simulink model "Copy_of_Controller"  (R2023a)
settings: Solver=FixedStepDiscrete  StartTime=0.0  StopTime=inf  FixedStep=0.001  RelTol=1e-3  EnableMultiTasking=on
undefined symbols (not defined in the file or in its folder): C, den_d, Discrete, K, K_down, num_d, sys_d, sys_d_down, Time
libraries: simulink x12, quarc_library x4, eeGeneralControl x4, ctrlSharedLib x2, simulink_extras x1
settings Model: SimulationMode=external  ExtModeTrigType=signal  ExtModeTrigDuration=60000  ExtModeTrigDirection=either  ExtModeTrigLevel=0.500000  Creator=colegiusto  LastModifiedBy=colegiusto
settings SolverCC: PositivePriorityOrder=on
settings RTWCC: Description=QUARC Win64 Target Using Toolchain  SystemTargetFile=quarc_win64.tlc  Toolchain=QUARC win64 | nmake (64-bit Windows)  BuildConfiguration=Faster Runs
settings STFCustomTargetCC: TargetLangStandard=C89/C90 (ANSI)  SystemTargetFile=quarc_win64.tlc
settings GRTTargetCC: TargetLangStandard=C89/C90 (ANSI)  ParMdlRefBuildCompliant=off  CompOptLevelCompliant=off  CombineOutputUpdateFcns=off  MatFileLogging=off  CPPClassGenCompliant=off  GRTInterface=on  ExtMode=on  ExtModeMexFile=quarc_comm

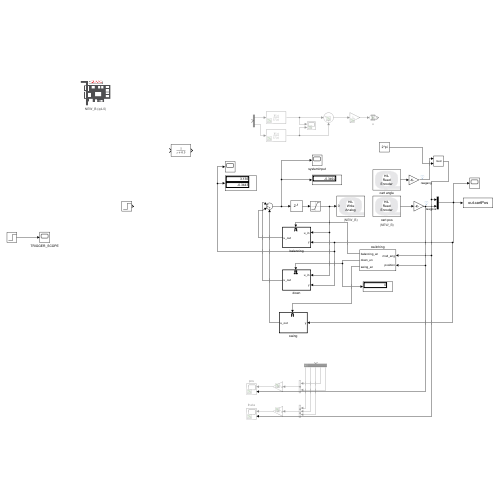
[thumbnail: Simulink's stored preview of the top-level diagram]
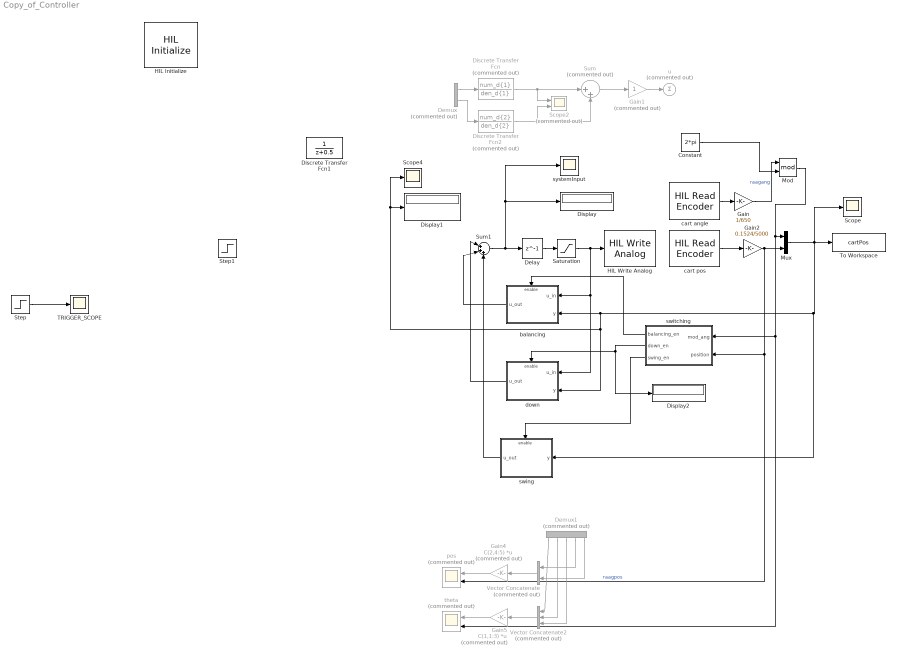
== system Copy_of_Controller ==
  Constant : Constant  Value=2*pi
  Delay : Delay  DelayLength=1
  Demux : Demux  Commented=on  Outputs=2
  Demux1 : Demux  Commented=on  Outputs=5
  Discrete Transfer Fcn : DiscreteTransferFcn  Commented=on  Numerator=num_d{1}  Denominator=den_d{1}  SampleTime=0.001
  Discrete Transfer Fcn1 : DiscreteTransferFcn
  Discrete Transfer Fcn2 : DiscreteTransferFcn  Commented=on  Numerator=num_d{2}  Denominator=den_d{2}  SampleTime=0.001
  Display : Display
  Display1 : Display
  Display2 : Display
  Gain : Gain  Gain=1/650
  Gain1 : Gain  Commented=on
  Gain2 : Gain  Gain=0.1524/5000
  Gain4 : Gain  Commented=on  Gain=C(2,4:5)  Multiplication=Matrix(K*u)
  Gain5 : Gain  Commented=on  Gain=C(1,1:3)  Multiplication=Matrix(K*u)
  HIL Initialize : quarc_library/Data Acquisition/Generic/Configuration/HIL Initialize  object_name=NEW_B  board_type=q4  board_number=0  board_options=""  exclusive=off  active=on  hardware_clocks=[0:1]  clock_modes=[0 0]  initial_clock_frequencies=[]  set_clock_params_at_start=on  set_clock_params_at_switch_in=off  set_clock_frequencies_at_start=off  set_clock_frequencies_at_switch_in=off  analog_input_channels=[0:3]  analog_input_configurations=[]  analog_input_maximums=10  analog_input_minimums=-10  set_analog_input_params_at_start=off  set_analog_input_params_at_switch_in=off  analog_output_channels=[0:3]  analog_output_maximums=[10]  analog_output_minimums=[-10]  initial_analog_outputs=[0]  final_analog_outputs=[0]  watchdog_analog_outputs=0  set_analog_output_params_at_start=on  set_analog_output_params_at_switch_in=off  set_analog_outputs_at_start=on  set_analog_outputs_at_switch_in=off  set_analog_outputs_at_terminate=on  set_analog_outputs_at_switch_out=off  set_analog_outputs_on_watchdog=off  digital_input_channels=[]  digital_output_channels=[]  digital_output_configuration=[]  initial_digital_outputs=[1]  final_digital_outputs=[1]  watchdog_digital_outputs=[2]  set_digital_output_params_at_start=off  set_digital_output_params_at_switch_in=off  set_digital_outputs_at_start=on  set_digital_outputs_at_switch_in=off  set_digital_outputs_at_terminate=on  set_digital_outputs_at_switch_out=off  set_digital_outputs_on_watchdog=off  encoder_channels=[0:3]  quadrature=[4]  encoder_filter_frequency=(1/60e-9)/1  initial_encoder_counts=[0]  set_encoder_params_at_start=on  set_encoder_params_at_switch_in=off  set_encoder_counts_at_start=on  set_encoder_counts_at_switch_in=off  pwm_channels=[]  pwm_modes=[0]  pwm_frequency=(1/60e-9)/1024  pwm_configuration=[]  pwm_alignment=[]  pwm_polarity=[]  pwm_leading_deadband=[]  pwm_trailing_deadband=[]  initial_pwm_outputs=[0]  final_pwm_outputs=[0]  watchdog_pwm_outputs=[]  set_pwm_params_at_start=on  set_pwm_params_at_switch_in=off  set_pwm_outputs_at_start=on  set_pwm_outputs_at_switch_in=off  set_pwm_outputs_at_terminate=on  set_pwm_outputs_at_switch_out=off  set_pwm_outputs_on_watchdog=off  other_output_channels=[]  initial_other_outputs=[]  final_other_outputs=[]  watchdog_other_outputs=[]  set_other_outputs_at_start=off  set_other_outputs_at_switch_in=off  set_other_outputs_at_terminate=off  set_other_outputs_at_switch_out=off  set_other_outputs_on_watchdog=off
  HIL Write Analog : quarc_library/Data Acquisition/Generic/Immediate I//O/HIL Write Analog  object_name=NEW_B  channels=0  sample_time=0.001  active=off  vector_input=off
  Mod : Math  Operator=mod
  Mux : Mux  Inputs=2
  Saturation : Saturate  UpperLimit=5  LowerLimit=-5
  Scope : Scope
  Scope2 : Scope  Commented=on  NumInputPorts=2
  Scope4 : Scope
  Step : Step  Time=0.001  SampleTime=0
  Step1 : Step  After=0.3  SampleTime=0
  Sum : Sum  Commented=on  Inputs=|++
  Sum1 : Sum  Inputs=|+++
  TRIGGER_SCOPE : Scope
  To Workspace : ToWorkspace  VariableName=cartPos  SaveFormat=Structure With Time  SampleTime=-1
  Vector Concatenate : Concatenate  Commented=on
  Vector Concatenate2 : Concatenate  Commented=on  NumInputs=3
  balancing : Subsystem
  cart angle : quarc_library/Data Acquisition/Generic/Immediate I//O/HIL Read Encoder  object_name=NEW_B  channels=3  sample_time=0.001  active=on  vector_output=on  data_type_mode=Inherit via back propagation  data_type=double
  cart pos : quarc_library/Data Acquisition/Generic/Immediate I//O/HIL Read Encoder  object_name=NEW_B  channels=2  sample_time=0.001  active=on  vector_output=on  data_type_mode=Inherit via back propagation  data_type=double
  down : Subsystem
  pos : Scope  Commented=on  NumInputPorts=2
  swing : Subsystem
  switching : Subsystem
  systemInput : Scope
  theta : Scope  Commented=on  NumInputPorts=2
  u : Sum  Commented=on  Inputs=+
  wires:
  cart angle/1 -> Gain/1
  Step/1 -> TRIGGER_SCOPE/1
  Gain/1 -> Mod/1  "raagang"
  Mux/1 -> swing/1(y), balancing/2(y), down/2(y), Scope4/1, Display1/1, To Workspace/1, Scope/1
  Saturation/1 -> balancing/1(u_in), down/1(u_in), HIL Write Analog/1
  cart pos/1 -> Gain2/1
  Gain2/1 -> Mux/2, switching/2(position), pos/2  "raagpos"
  Demux/1 -> Discrete Transfer Fcn/1
  Demux/2 -> Discrete Transfer Fcn2/1
  Sum/1 -> Gain1/1
  Discrete Transfer Fcn2/1 -> Sum/2, Scope2/2
  Discrete Transfer Fcn/1 -> Sum/1, Scope2/1
  Gain1/1 -> u/1
  Demux1/4 -> Vector Concatenate/1
  Demux1/5 -> Vector Concatenate/2
  Vector Concatenate/1 -> Gain4/1
  Demux1/1 -> Vector Concatenate2/1
  Demux1/2 -> Vector Concatenate2/2
  Demux1/3 -> Vector Concatenate2/3
  Vector Concatenate2/1 -> Gain5/1
  Gain4/1 -> pos/1
  Gain5/1 -> theta/1
  Constant/1 -> Mod/2
  Mod/1 -> theta/2, switching/1(mod_ang), Mux/1
  Delay/1 -> Saturation/1
  switching/1(balancing_en) -> balancing/Enable
  switching/2(down_en) -> Display2/1, down/Enable
  balancing/1(u_out) -> Sum1/2
  Sum1/1 -> systemInput/1, Display/1, Delay/1
  switching/3(swing_en) -> swing/Enable
  swing/1(u_out) -> Sum1/3
  down/1(u_out) -> Sum1/1

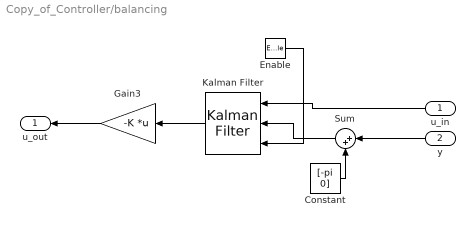
== system Copy_of_Controller/balancing ==
  u_in : Inport
  y : Inport  Port=2
  Enable : EnablePort  StatesWhenEnabling=reset  ShowOutputPort=on
  Constant : Constant  Value=[-pi 0]
  Gain3 : Gain  Gain=-K  Multiplication=Matrix(K*u)
  Kalman Filter : ctrlSharedLib/Kalman Filter  TimeDomain=Discrete-Time  UseCurrentEstimator=on  ModelSource=Individual A, B, C, D matrices  ModelSourceVariable=ss(0.95,1,1,0,1)  A=sys_d.A  B=sys_d.B  C=sys_d.C  D=sys_d.D  NumberOfStates=1  NumberOfInputs=1  NumberOfOutputs=1  InitialEstimateSource=Dialog  X0=0  P0=10  UseK=off  UseGH=off  NumberOfProcessNoiseInputs=1  G=1  TimeInvariantG=on  H=0  TimeInvariantH=on  Q=1  TimeInvariantQ=on  R=10  TimeInvariantR=on  N=0  TimeInvariantN=on  AddInputPort=on  AddEnablePort=off  ExternalReset=Rising  OutputEstimatedY=off  OutputP=off  Ts=0.001
  Sum : Sum  Inputs=|++
  u_out : Outport  OutputWhenDisabled=reset  InitialOutput=[0]
  wires:
  Kalman Filter/1 -> Gain3/1
  u_in/1 -> Kalman Filter/1
  Gain3/1 -> u_out/1
  y/1 -> Sum/1
  Constant/1 -> Sum/2
  Sum/1 -> Kalman Filter/2
  Enable/1 -> Kalman Filter/3

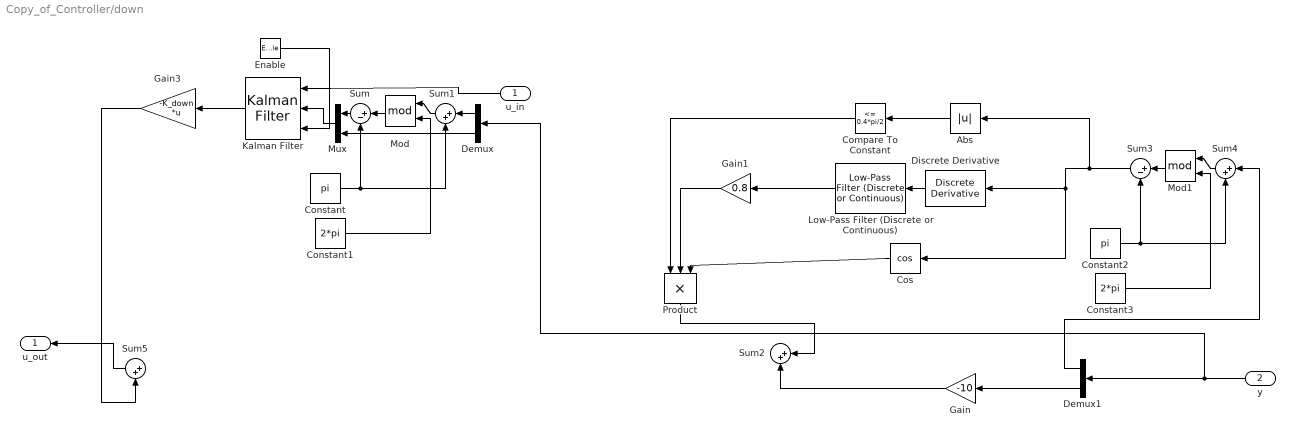
== system Copy_of_Controller/down ==
  u_in : Inport
  y : Inport  Port=2
  Enable : EnablePort  StatesWhenEnabling=reset  ShowOutputPort=on
  Abs : Abs  SaturateOnIntegerOverflow=off
  Compare To Constant : simulink/Logic and Bit Operations/Compare To Constant  relop=<=  const=0.4*pi/2  OutDataTypeStr=boolean
  Constant : Constant  Value=pi
  Constant1 : Constant  Value=2*pi
  Constant2 : Constant  Value=pi
  Constant3 : Constant  Value=2*pi
  Cos : Trigonometry  Operator=cos
  Demux : Demux  Outputs=2
  Demux1 : Demux  Outputs=2
  Discrete Derivative : simulink/Discrete/Discrete Derivative  gainval=1.0  ICPrevScaledInput=0.0  OutMin=[]  OutMax=[]  OutDataType=fixdt(1, 16)  OutScaling=2^-10  DoSatur=off
  Gain : Gain  Gain=-10
  Gain1 : Gain  Gain=0.8
  Gain3 : Gain  Gain=-K_down  Multiplication=Matrix(K*u)
  Kalman Filter : ctrlSharedLib/Kalman Filter  TimeDomain=Discrete-Time  UseCurrentEstimator=on  ModelSource=Individual A, B, C, D matrices  ModelSourceVariable=ss(0.95,1,1,0,1)  A=sys_d_down.A  B=sys_d_down.B  C=sys_d_down.C  D=sys_d_down.D  NumberOfStates=1  NumberOfInputs=1  NumberOfOutputs=1  InitialEstimateSource=Dialog  X0=0  P0=10  UseK=off  UseGH=off  NumberOfProcessNoiseInputs=1  G=1  TimeInvariantG=on  H=0  TimeInvariantH=on  Q=1  TimeInvariantQ=on  R=10  TimeInvariantR=on  N=0  TimeInvariantN=on  AddInputPort=on  AddEnablePort=off  ExternalReset=Rising  OutputEstimatedY=off  OutputP=off  Ts=0.001
  Low-Pass Filter (Discrete or Continuous) : eeGeneralControl/Low-Pass Filter (Discrete or Continuous)  K=1  T=0.01  B=inf  A=-inf  init_option=Inherited from block input  x0=0  Ts=-1
  Mod : Math  Operator=mod
  Mod1 : Math  Operator=mod
  Mux : Mux  Inputs=2
  Product : Product  Inputs=3
  Sum : Sum  Inputs=|+-
  Sum{1..2,4..5} (4 alike) : Sum  Inputs=|++
  Sum3 : Sum  Inputs=|+-
  u_out : Outport  OutputWhenDisabled=reset  InitialOutput=[0]
  wires:
  Kalman Filter/1 -> Gain3/1
  u_in/1 -> Kalman Filter/1
  Demux/2 -> Mux/2
  Mux/1 -> Kalman Filter/2
  Demux/1 -> Sum1/1
  Mod/1 -> Sum/1
  Sum1/1 -> Mod/1
  Constant/1 -> Sum1/2, Sum/2
  Constant1/1 -> Mod/2
  Sum/1 -> Mux/1
  Constant3/1 -> Mod1/2
  Product/1 -> Sum2/1
  Gain1/1 -> Product/2
  Cos/1 -> Product/3
  Sum3/1 -> Abs/1, Cos/1, Discrete Derivative/1
  Abs/1 -> Compare To Constant/1
  Demux1/2 -> Gain/1
  Gain/1 -> Sum2/2
  Constant2/1 -> Sum4/2, Sum3/2
  Demux1/1 -> Sum4/1
  Sum4/1 -> Mod1/1
  Compare To Constant/1 -> Product/1
  Discrete Derivative/1 -> Low-Pass Filter (Discrete or Continuous)/1
  Mod1/1 -> Sum3/1
  y/1 -> Demux/1, Demux1/1
  Low-Pass Filter (Discrete or Continuous)/1 -> Gain1/1
  Gain3/1 -> Sum5/2
  Sum5/1 -> u_out/1
  Enable/1 -> Kalman Filter/3

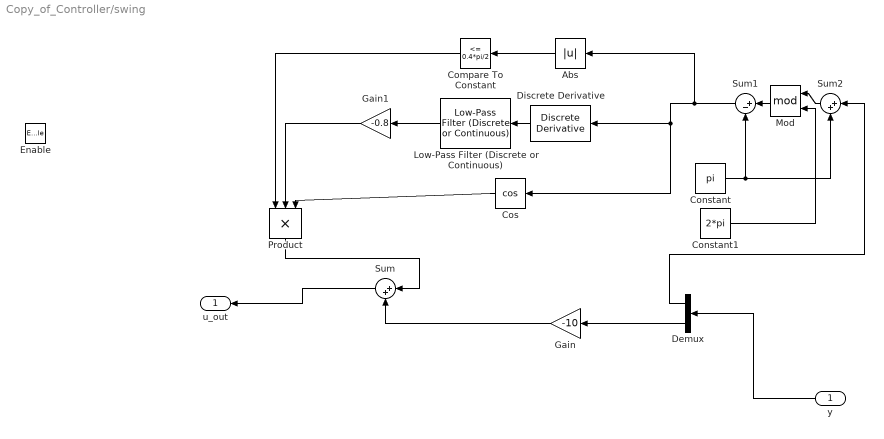
== system Copy_of_Controller/swing ==
  y : Inport
  Enable : EnablePort  StatesWhenEnabling=reset
  Abs : Abs  SaturateOnIntegerOverflow=off
  Compare To Constant : simulink/Logic and Bit Operations/Compare To Constant  relop=<=  const=0.4*pi/2  OutDataTypeStr=boolean
  Constant : Constant  Value=pi
  Constant1 : Constant  Value=2*pi
  Cos : Trigonometry  Operator=cos
  Demux : Demux  Outputs=2
  Discrete Derivative : simulink/Discrete/Discrete Derivative  gainval=1.0  ICPrevScaledInput=0.0  OutMin=[]  OutMax=[]  OutDataType=fixdt(1, 16)  OutScaling=2^-10  DoSatur=off
  Gain : Gain  Gain=-10
  Gain1 : Gain  Gain=-0.8
  Low-Pass Filter (Discrete or Continuous) : eeGeneralControl/Low-Pass Filter (Discrete or Continuous)  K=1  T=0.01  B=inf  A=-inf  init_option=Inherited from block input  x0=0  Ts=-1
  Mod : Math  Operator=mod
  Product : Product  Inputs=3
  Sum : Sum  Inputs=|++
  Sum1 : Sum  Inputs=|+-
  Sum2 : Sum  Inputs=|++
  u_out : Outport  OutputWhenDisabled=reset  InitialOutput=[0]
  wires:
  y/1 -> Demux/1
  Sum/1 -> u_out/1
  Demux/2 -> Gain/1
  Gain/1 -> Sum/2
  Demux/1 -> Sum2/1
  Discrete Derivative/1 -> Low-Pass Filter (Discrete or Continuous)/1
  Low-Pass Filter (Discrete or Continuous)/1 -> Gain1/1
  Constant/1 -> Sum2/2, Sum1/2
  Constant1/1 -> Mod/2
  Mod/1 -> Sum1/1
  Sum2/1 -> Mod/1
  Sum1/1 -> Abs/1, Cos/1, Discrete Derivative/1
  Gain1/1 -> Product/2
  Product/1 -> Sum/1
  Abs/1 -> Compare To Constant/1
  Compare To Constant/1 -> Product/1
  Cos/1 -> Product/3

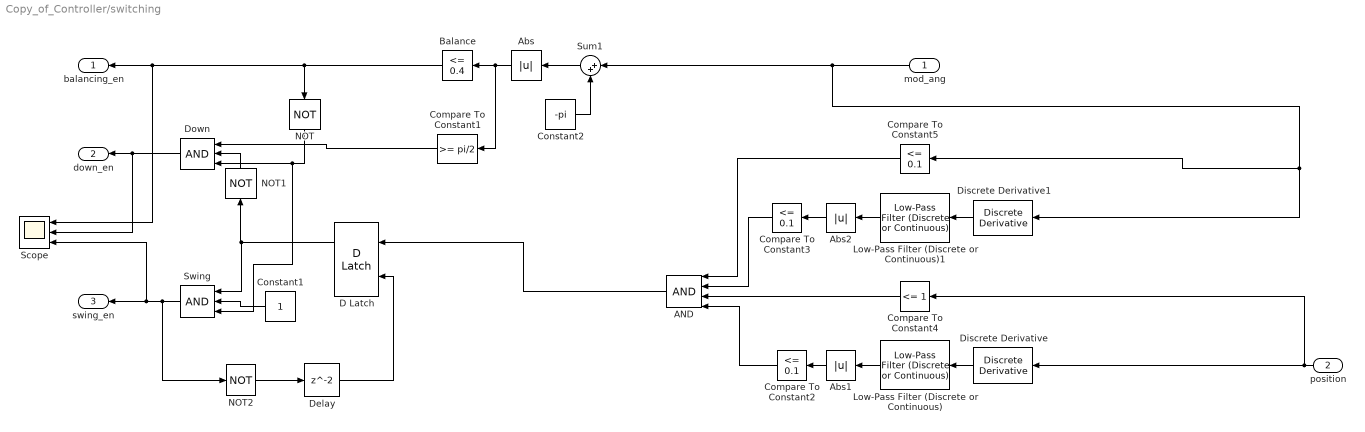
== system Copy_of_Controller/switching ==
  mod_ang : Inport
  position : Inport  Port=2
  AND : Logic  Inputs=4  IconShape=distinctive  AllPortsSameDT=off  OutDataTypeStr=boolean
  Abs : Abs  SaturateOnIntegerOverflow=off
  Abs1 : Abs  SaturateOnIntegerOverflow=off
  Abs2 : Abs  SaturateOnIntegerOverflow=off
  Balance : simulink/Logic and Bit Operations/Compare To Constant  relop=<=  const=0.4  OutDataTypeStr=boolean
  Compare To Constant1 : simulink/Logic and Bit Operations/Compare To Constant  relop=>=  const=pi/2  OutDataTypeStr=boolean
  Compare To Constant2 : simulink/Logic and Bit Operations/Compare To Constant  relop=<=  const=0.1  OutDataTypeStr=boolean
  Compare To Constant3 : simulink/Logic and Bit Operations/Compare To Constant  relop=<=  const=0.1  OutDataTypeStr=boolean
  Compare To Constant4 : simulink/Logic and Bit Operations/Compare To Constant  relop=<=  const=1  OutDataTypeStr=boolean
  Compare To Constant5 : simulink/Logic and Bit Operations/Compare To Constant  relop=<=  const=0.1  OutDataTypeStr=boolean
  Constant1 : Constant
  Constant2 : Constant  Value=-pi
  D Latch : simulink_extras/Flip Flops/D Latch
  Delay : Delay
  Discrete Derivative : simulink/Discrete/Discrete Derivative  gainval=1.0  ICPrevScaledInput=0.0  OutMin=[]  OutMax=[]  OutDataType=fixdt(1, 16)  OutScaling=2^-10  DoSatur=off
  Discrete Derivative1 : simulink/Discrete/Discrete Derivative  gainval=1.0  ICPrevScaledInput=0.0  OutMin=[]  OutMax=[]  OutDataType=fixdt(1, 16)  OutScaling=2^-10  DoSatur=off
  Down : Logic  Inputs=3  IconShape=distinctive  AllPortsSameDT=off  OutDataTypeStr=boolean
  Low-Pass Filter (Discrete or Continuous) : eeGeneralControl/Low-Pass Filter (Discrete or Continuous)  K=1  T=1/100  B=inf  A=-inf  init_option=Inherited from block input  x0=0  Ts=0.001
  Low-Pass Filter (Discrete or Continuous)1 : eeGeneralControl/Low-Pass Filter (Discrete or Continuous)  K=1  T=1/100  B=inf  A=-inf  init_option=Inherited from block input  x0=0  Ts=0.001
  NOT : Logic  Operator=NOT  IconShape=distinctive  AllPortsSameDT=off  OutDataTypeStr=boolean
  NOT1 : Logic  Operator=NOT  IconShape=distinctive  AllPortsSameDT=off  OutDataTypeStr=boolean
  NOT2 : Logic  Operator=NOT  IconShape=distinctive  AllPortsSameDT=off  OutDataTypeStr=boolean
  Scope : Scope  NumInputPorts=3
  Sum1 : Sum  Inputs=|++
  Swing : Logic  Inputs=3  IconShape=distinctive  AllPortsSameDT=off  OutDataTypeStr=boolean
  balancing_en : Outport
  down_en : Outport  Port=2
  swing_en : Outport  Port=3
  wires:
  Sum1/1 -> Abs/1
  Abs/1 -> Compare To Constant1/1, Balance/1
  Constant2/1 -> Sum1/2
  mod_ang/1 -> Compare To Constant5/1, Discrete Derivative1/1, Sum1/1
  Balance/1 -> NOT/1, Scope/1, balancing_en/1
  position/1 -> Compare To Constant4/1, Discrete Derivative/1
  Discrete Derivative/1 -> Low-Pass Filter (Discrete or Continuous)/1
  Low-Pass Filter (Discrete or Continuous)/1 -> Abs1/1
  Abs1/1 -> Compare To Constant2/1
  Abs2/1 -> Compare To Constant3/1
  Low-Pass Filter (Discrete or Continuous)1/1 -> Abs2/1
  Discrete Derivative1/1 -> Low-Pass Filter (Discrete or Continuous)1/1
  Compare To Constant5/1 -> AND/1
  Compare To Constant3/1 -> AND/2
  Compare To Constant4/1 -> AND/3
  Compare To Constant2/1 -> AND/4
  Constant1/1 -> Swing/2
  Swing/1 -> NOT2/1, Scope/3, swing_en/1
  Compare To Constant1/1 -> Down/1
  Down/1 -> Scope/2, down_en/1
  NOT1/1 -> Down/2
  NOT/1 -> Swing/3, Down/3
  D Latch/1 -> Swing/1, NOT1/1
  AND/1 -> D Latch/1
  NOT2/1 -> Delay/1
  Delay/1 -> D Latch/2
